simulink model "pm_p4_motor_controladoresIndividuales"  (R2019b)
settings: Solver=VariableStepAuto  StartTime=0.0  StopTime=3.0  RelTol=1e-3
settings Model: Creator=robotica  LastModifiedBy=arlette
settings DataIOCC: ReturnWorkspaceOutputs=off
settings DebuggingCC: ArithmeticOperatorsInVariantConditions=warning
settings SFSimCC: SimUseLocalCustomCode=off  CustomCodeUndefinedFunction=UseInterfaceOnly
settings RTWCC: RTWUseLocalCustomCode=off
settings CodeAppCC: StateflowObjectComments=on

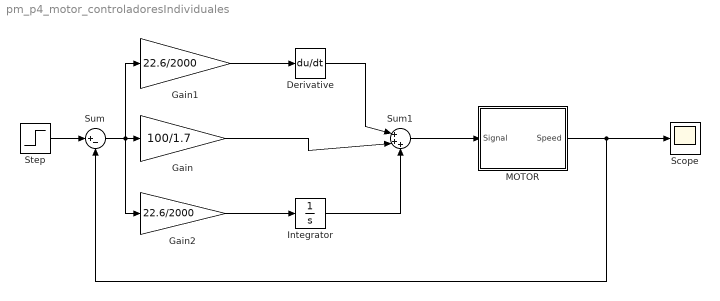
== system pm_p4_motor_controladoresIndividuales ==
  Derivative : Derivative
  Gain : Gain  Gain=100/1.7
  Gain1 : Gain  Gain=22.6/2000
  Gain2 : Gain  Gain=22.6/2000
  Integrator : Integrator
  MOTOR : Subsystem
  Scope : Scope
  Step : Step  SampleTime=0
  Sum : Sum  Inputs=|+-
  Sum1 : Sum  Inputs=|+++
  wires:
  Step/1 -> Sum/1
  Sum/1 -> Gain2/1, Gain/1, Gain1/1
  Gain2/1 -> Integrator/1
  Gain1/1 -> Derivative/1
  Derivative/1 -> Sum1/1
  Gain/1 -> Sum1/2
  Integrator/1 -> Sum1/3
  Sum1/1 -> MOTOR/1(Signal)
  MOTOR/1(Speed) -> Sum/2, Scope/1

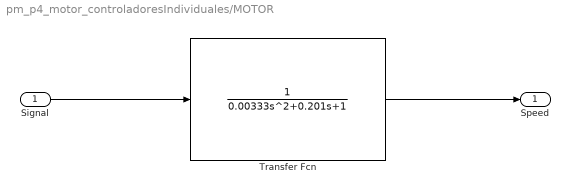
== system pm_p4_motor_controladoresIndividuales/MOTOR ==
  Signal : Inport
  Transfer Fcn : TransferFcn  Denominator=[0.00333 0.201 1]
  Speed : Outport  VectorParamsAs1DForOutWhenUnconnected=off
  wires:
  Transfer Fcn/1 -> Speed/1
  Signal/1 -> Transfer Fcn/1
